simulink model "prof_eq"  (R2017b)
settings: Solver=VariableStepAuto  StartTime=0.0  StopTime=1200  RelTol=1e-6
values from neighbouring files (symbols this model uses):
  xi = [v_ini, gamma_ini, h_ini, phi_ini, theta_ini, q_ini]    [load_to_simulink.m]    (also in reentry_simulator.m)
undefined symbols (not defined in the file or in its folder): Atm, Mars, sim_params, Vehicle
settings Model: Creator=Administrateur  LastModifiedBy=Administrateur

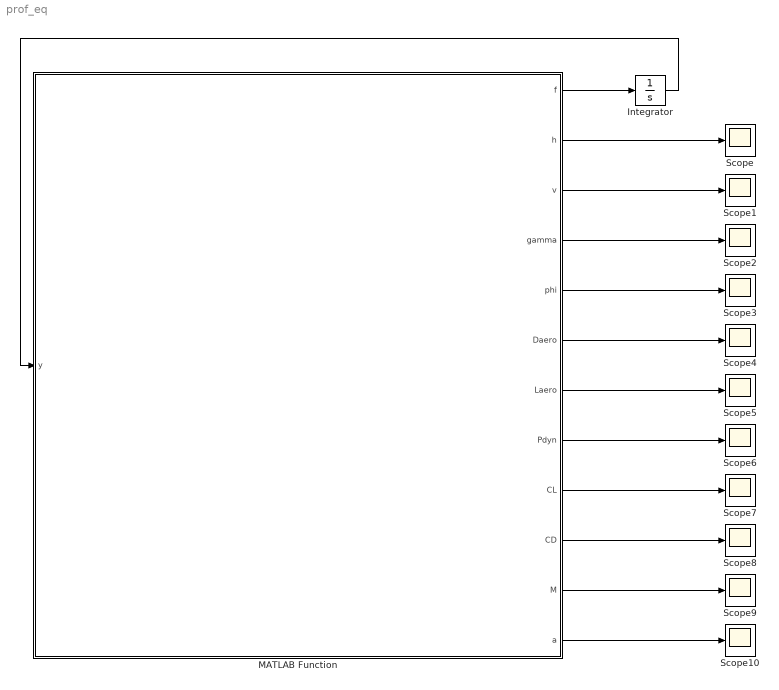
== system prof_eq ==
  Integrator : Integrator  InitialCondition=xi
  MATLAB Function : MATLAB Function  TreatAsAtomicUnit=on
  Scope{,1..10} (11 alike) : Scope
  wires:
  MATLAB Function/1(f) -> Integrator/1
  Integrator/1 -> MATLAB Function/1(y)
  MATLAB Function/2(h) -> Scope/1
  MATLAB Function/3(v) -> Scope1/1
  MATLAB Function/7(Laero) -> Scope5/1
  MATLAB Function/6(Daero) -> Scope4/1
  MATLAB Function/5(phi) -> Scope3/1
  MATLAB Function/4(gamma) -> Scope2/1
  MATLAB Function/8(Pdyn) -> Scope6/1
  MATLAB Function/9(CL) -> Scope7/1
  MATLAB Function/10(CD) -> Scope8/1
  MATLAB Function/11(M) -> Scope9/1
  MATLAB Function/12(a) -> Scope10/1

== matlab function prof_eq/MATLAB Function ==
  data: y input; f output; h output; v output; Mars parameter; Atm parameter; Vehicle parameter; sim_params parameter; gamma output; phi output; Daero output; Laero output; Pdyn output; CL output; CD output; M output; a output
function [f, h, v, gamma, phi, Daero, Laero, Pdyn, CL, CD, M, a] = Dynamics(y, Mars, Atm, Vehicle, sim_params)
    v = y(1);
    gamma = y(2);
    h = y(3);
    phi = y(4);
    theta = y(5);
    q = y(6);
    % m = y(5) To be implemented
    f = [0; 0; 0; 0; 0; 0];
    % Intermediate calculation
    r = h + Mars.radius * 1000;
    g = Mars.mu * 1e9 / r^2; % m/s^2 - Gravitationnal acceleration at r
    if h > 120000
        rho = 0;
    else
        rho =  Atm.rho0 * exp(-h/Atm.hs);
    end
    Pdyn = (1/2) * rho * (v^2 + 0.241^2); % Dynamic pressure

    
    if h < 10000
        t = -1.019e-11 * h.^3 + 1.349e-08 * h.^2 +...
            -1.958e-05 * h.^1 + 214; % K - Temperature
    elseif h >= 10000 && h <= 70000
        t = 2.845e-18 * h.^4 + -4.139e-13 * h.^3 + ...
              3.048e-08 * h.^2 -0.002304 * h.^1 + ...
              225.2; % K - Temperature
    elseif h > 70000 && h <= 100000
        t = 139; % K - Temperature
    else
        t = 0.001035 * h + 35.52; % K - Temperature
    end
    speed = sqrt(Atm.gamma * Atm.R * t);
    M = v / speed;
    alpha = deg2rad(-5);
    
    CA = CASimulink(M, alpha);
    CN = CNSimulink(M, alpha);
    
    CD = CA;
    CL = CD * (-0.016 * rad2deg(alpha));
     
    Daero = Pdyn * Vehicle.S * CD;
    Laero = Pdyn * Vehicle.S * CL;
    
    if (h <= sim_params.parachute_at || M < sim_params.parachute_mach)
        Daero = Vehicle.Parachute.CD .* ((rho .* v.^2) / 2) * Vehicle.Parachute.S;
        Laero = 0;
    end
    
    if (h <= 0)
        f(1) = 0;
    elseif (h <= sim_params.parachute_at || M < sim_params.parachute_mach)
        f(1) = (-Daero) / Vehicle.mass + g;
    else
        f(1) = (-Daero) / Vehicle.mass + g*sin(gamma);
    end
    a = f(1);
    
    if(h <= 0)
        f(2) = 0;
    else
        f(2) = (Laero/Vehicle.mass + (g ./ v - (v.^2/r))*cos(gamma));
    end
    
    if (h <= 0)
        f(3) = 0;
    elseif((h <= sim_params.parachute_at) || M < sim_params.parachute_mach)
        f(3) = -v;
    else
        f(3) = v * sin(gamma);
    end
    
    if (h <= 0)
        f(4) = 0;
    else
        f(4) = v/r * cos(gamma);
    end
    f(5) = 0;
    f(6) = 0;
    
    f = f(:);
end
